simulink model "PID_Discrete"  (R2021b)
settings: Solver=VariableStepAuto  StartTime=0.0  StopTime=5  RelTol=1e-3  EnableMultiTasking=on
libraries: dspsrcs4 x3, simulink_extras x2, dspsigops x2, slpidlib x1, dsparch4 x1
settings Model: Creator=JelleKomen  LastModifiedBy=JelleKomen
settings DebuggingCC: SignalRangeChecking=warning

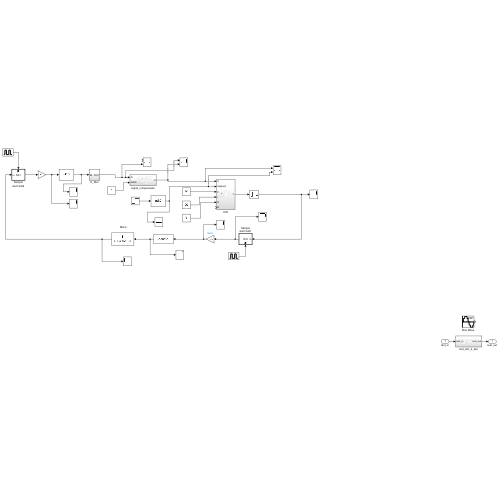
[thumbnail: Simulink's stored preview of the top-level diagram]
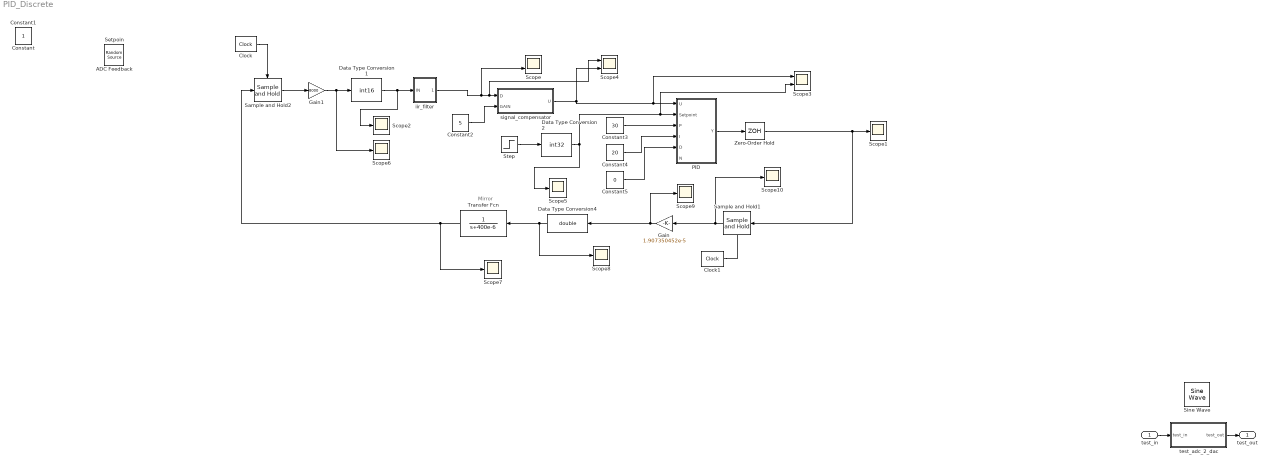
== system PID_Discrete ==
  note: Mirror
  test_in : Inport
  Clock : simulink_extras/Flip Flops/Clock  period=100e-9
  Clock1 : simulink_extras/Flip Flops/Clock  period=1e-6
  Constant2 : Constant  Value=5  OutDataTypeStr=uint8
  Constant3 : Constant  Value=30  OutDataTypeStr=int32
  Constant4 : Constant  Value=20  OutDataTypeStr=int32
  Constant5 : Constant  Value=0  OutDataTypeStr=int32
  Data Type Conversion1 : DataTypeConversion  OutDataTypeStr=int16
  Data Type Conversion2 : DataTypeConversion  OutDataTypeStr=int32
  Data Type Conversion4 : DataTypeConversion  OutDataTypeStr=double  SaturateOnIntegerOverflow=on
  Gain : Gain  Gain=1.907350452e-5
  Gain1 : Gain  Gain=8000
  PID : Subsystem
  Sample and Hold1 : dspsigops/Sample and Hold  trig=Rising edge  initCond=0  latchinput=off
  Sample and Hold2 : dspsigops/Sample and Hold  trig=Rising edge  initCond=0  latchinput=off
  Scope : Scope  NumInputPorts=2
  Scope{1..2,5..10} (8 alike) : Scope
  Scope3 : Scope  NumInputPorts=2
  Scope4 : Scope  NumInputPorts=2
  Sine Wave : dspsrcs4/Sine Wave  Amplitude=32767  Frequency=1e3  Phase=0  SampleMode=Discrete  OutComplex=Real  CompMethod=Table lookup  TableSize=Speed  SampleTime=1/10e6  SamplesPerFrame=1  ResetState=Restart at time zero  OutputFrames=off  dataType=Fixed-point  wordLen=16  udDataType=sfix(16)  fracBitsMode=User-defined  numFracBits=0  OutDataTypeStr=fixdt(1,16,0)  LastOutDataTypeStr=fixdt(1,16,0)
  Step : Step  Time=0.001  After=8000  SampleTime=0
  Transfer Fcn : TransferFcn  Denominator=[1 400e-6]
  Zero-Order Hold : ZeroOrderHold  SampleTime=-1
  iir_filter : Subsystem
  signal_compensator : Subsystem
  test_adc_2_dac : Subsystem
  test_out : Outport  VectorParamsAs1DForOutWhenUnconnected=off
  ADC Feedback : dspsrcs4/Random Source  IOType=siggen  SrcType=Uniform  NormMethod=Ziggurat  CltLength=12  MinVal=0  MaxVal=1  MeanVal=0  VarVal=1  RepMode=Not repeatable  rawSeed=1  IsInherit=off  SampMode=Discrete  SampTime=1  SampFrame=1  DataType=Double  OutComplex=Real  OutputFrames=on
  Constant : Constant  IOType=siggen
  Constant1 : Constant  IOType=siggen
  Setpoin : dspsrcs4/Random Source  IOType=siggen  SrcType=Uniform  NormMethod=Ziggurat  CltLength=12  MinVal=0  MaxVal=1  MeanVal=0  VarVal=1  RepMode=Not repeatable  rawSeed=1  IsInherit=off  SampMode=Discrete  SampTime=1  SampFrame=1  DataType=Double  OutComplex=Real  OutputFrames=on
  wires:
  test_in/1 -> test_adc_2_dac/1(test_in)
  test_adc_2_dac/1(test_out) -> test_out/1
  Constant2/1 -> signal_compensator/2(GAIN)
  signal_compensator/1(U) -> Scope4/2, PID/1(U), Scope3/1
  Zero-Order Hold/1 -> Sample and Hold1/1, Scope1/1
  Sample and Hold1/1 -> Gain/1, Scope10/1
  Clock1/1 -> Sample and Hold1/Trigger
  Data Type Conversion4/1 -> Transfer Fcn/1, Scope8/1
  PID/1(Y) -> Zero-Order Hold/1
  Step/1 -> Data Type Conversion2/1
  Data Type Conversion2/1 -> Scope5/1, PID/2(Setpoint), Scope3/2
  Constant3/1 -> PID/3(P)
  Gain/1 -> Scope9/1, Data Type Conversion4/1
  Constant4/1 -> PID/4(I)
  Transfer Fcn/1 -> Sample and Hold2/1, Scope7/1
  Constant5/1 -> PID/5(D)
  iir_filter/1(OUT) -> Scope/2, Scope4/1, signal_compensator/1(D)
  Gain1/1 -> Scope6/1, Data Type Conversion1/1
  Data Type Conversion1/1 -> Scope2/1, iir_filter/1(IN)
  Sample and Hold2/1 -> Gain1/1
  Clock/1 -> Sample and Hold2/Trigger

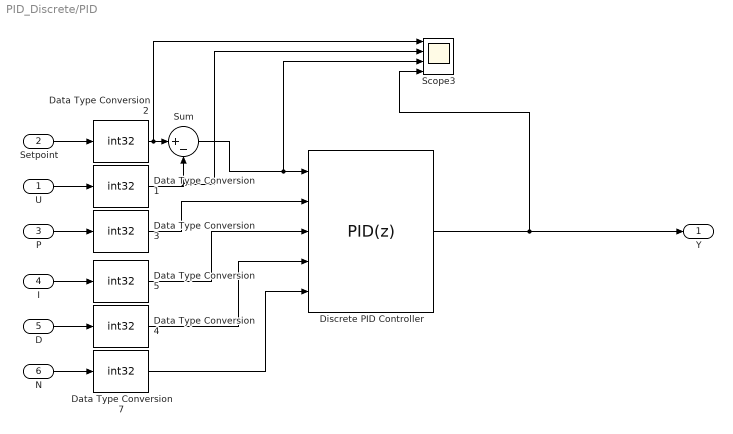
== system PID_Discrete/PID ==
  U : Inport  OutDataTypeStr=fixdt(1,20,0)
  Setpoint : Inport  Port=2  OutDataTypeStr=int32
  P : Inport  Port=3  OutDataTypeStr=int32
  I : Inport  Port=4  OutDataTypeStr=int32
  D : Inport  Port=5  OutDataTypeStr=int32
  N : Inport  Port=6  OutDataTypeStr=int32
  Data Type Conversion{1..5,7} (6 alike) : DataTypeConversion  OutDataTypeStr=int32  ConvertRealWorld=Stored Integer (SI)
  Discrete PID Controller : slpidlib/PID Controller  Controller=PID  Form=Parallel  TimeDomain=Discrete-time  UseExternalTs=off  SampleTime=-1  IntegratorMethod=Trapezoidal  FilterMethod=Forward Euler  ControllerParametersSource=external  P=1  I=1  D=0  UseFilter=on  N=100  TunerSelectOption=Transfer Function Based (PID Tuner App)  InitialConditionSource=internal  InitialConditionForIntegrator=0  InitialConditionForFilter=0  DifferentiatorICPrevScaledInput=0  ExternalReset=none  TrackingMode=off  Kt=1  LimitOutput=off  SatLimitsSource=internal  UpperSaturationLimit=inf  LowerSaturationLimit=-inf  LinearizeAsGain=off  AntiWindupMode=none  Kb=1  SaturateOnIntegerOverflow=on  PGainOutDataTypeStr=int32  PProdOutDataTypeStr=int32  POutMin=[]  POutMax=[]  IGainOutDataTypeStr=int32  IProdOutDataTypeStr=int32  IOutMin=[]  IOutMax=[]  DGainOutDataTypeStr=int32  DProdOutDataTypeStr=int32  DOutMin=[]  DOutMax=[]  NGainOutDataTypeStr=int32  NProdOutDataTypeStr=int32  NOutMin=[]  NOutMax=[]  SumOutDataTypeStr=int32  SumOutMin=[]  SumOutMax=[]  SaturationOutMin=[]  SaturationOutMax=[]  PParamMin=[]  PParamMax=[]  IParamMin=[]  IParamMax=[]  DParamMin=[]  DParamMax=[]  NParamMin=[]  NParamMax=[]  KbParamMin=[]  KbParamMax=[]  KtParamMin=[]  KtParamMax=[]  KbOutMin=[]  KbOutMax=[]  KtOutMin=[]  KtOutMax=[]  IntegratorOutDataTypeStr=int32  IntegratorOutMin=[]  IntegratorOutMax=[]  FilterOutDataTypeStr=int32  FilterOutMin=[]  FilterOutMax=[]  SumI1OutMin=[]  SumI1OutMax=[]  SumI2OutMin=[]  SumI2OutMax=[]  SumI3OutMin=[]  SumI3OutMax=[]  SumI4OutMin=[]  SumI4OutMax=[]  SumDOutDataTypeStr=int32  SumDOutMin=[]  SumDOutMax=[]  SumAccumDataTypeStr=int32  SumDAccumDataTypeStr=int32  DifferentiatorOutMin=[]  DifferentiatorOutMax=[]  FilterDiffOutCoefMin=[]  FilterDiffOutCoefMax=[]  ReciprocalOutMin=[]  ReciprocalOutMax=[]  SumDenOutMin=[]  SumDenOutMax=[]  SumNumOutMin=[]  SumNumOutMax=[]  DivideOutMin=[]  DivideOutMax=[]  UdiffTsProdOutMin=[]  UdiffTsProdOutMax=[]  NTsProdOutMin=[]  NTsProdOutMax=[]  UintegralTsProdOutMin=[]  UintegralTsProdOutMax=[]  UngainTsProdOutMin=[]  UngainTsProdOutMax=[]  IntegratorContinuousStateAttributes=''  IntegratorStateMustResolveToSignalObject=off  IntegratorRTWStateStorageClass=Auto  FilterContinuousStateAttributes=''  FilterStateMustResolveToSignalObject=off  FilterRTWStateStorageClass=Auto  ParallelPVariant=ExternalParameters  IdealPVariant=Disabled  IVariant=ExternalParameters  DVariant=ExternalParameters  IntegratorVariant=Discrete  SatVariant=Disabled  AWVariant=Passthrough  PCopyVariant=Disabled  TRVariant=Disabled  FdbkBlocksVariant=Forward  IdealPFdbkVariant=Disabled  SatFdbkVariant=Disabled  DerivativeFilterVariant=ForwardEulerFilter  NVariant=ExternalParameters  NCopyVariant=Disabled  FilterICVariant=InternalICsFilter  IntegratorICVariant=InternalICs  ExternalResetVariant=Disabled  TRSumVariant=Passthrough  SumFdbkVariant=Disabled  SumVariant=Sum_PID  TsampFilterVariant=InternalTs  TsampNgainVariant=Passthrough  TsampIntegralVariant=Passthrough  ExternalSaturationOutDataTypeStr=Inherit: Same as second input
      settings: LockScale=on
  Scope3 : Scope  NumInputPorts=4
  Sum : Sum  Inputs=|+-
  Y : Outport  OutDataTypeStr=fixdt(1,20,0)
  wires:
  U/1 -> Data Type Conversion1/1
  Data Type Conversion1/1 -> Scope3/2, Sum/2
  Data Type Conversion2/1 -> Scope3/1, Sum/1
  Setpoint/1 -> Data Type Conversion2/1
  P/1 -> Data Type Conversion3/1
  I/1 -> Data Type Conversion5/1
  D/1 -> Data Type Conversion4/1
  N/1 -> Data Type Conversion7/1
  Data Type Conversion3/1 -> Discrete PID Controller/2
  Data Type Conversion5/1 -> Discrete PID Controller/3
  Data Type Conversion4/1 -> Discrete PID Controller/4
  Data Type Conversion7/1 -> Discrete PID Controller/5
  Sum/1 -> Scope3/3, Discrete PID Controller/1
  Discrete PID Controller/1 -> Scope3/4, Y/1

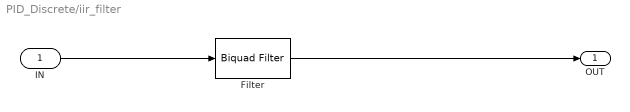
== system PID_Discrete/iir_filter ==
  IN : Inport  OutDataTypeStr=int16
  Filter : dsparch4/Biquad Filter  Tag=BlockMethodSubSystem  FilterSource=Dialog parameters  CoeffSource=Specify via dialog  FilterObject=BQF  IIRFiltStruct=Direct form II  BiQuadCoeffs=[1 2 1 1 -1.82450807943703452 0.904911483717982801;1 2 1 1 -1.67485327803320683 0.748661613958212513;1 2 1 1 -1.56987983878511672 0.639062148676173392;1 2 1 1 -1.50818165903315937 0.574645020323272693;1 1 0 1 -0.743936712675994705 0]  ScaleValues=[0.0201008510702371176;0.0184520839812514388;0.0172955774727642196;0.0166158403225283718;0.128031643662002703;1]  IC=0  ICnum=0  ICden=0  a0Flag=Warning  optimizeScaleValues=on  ScaleValueMode=Specify via input port (g)  InputProcessing=Columns as channels (frame based)  roundingMode=Floor  overflowMode=on  scaleValueFracLength=14  denProdOutputFracLength=30  denAccumFracLength=30  secondMemoryFracLength=15
  OUT : Outport  OutDataTypeStr=int16
  wires:
  IN/1 -> Filter/1
  Filter/1 -> OUT/1

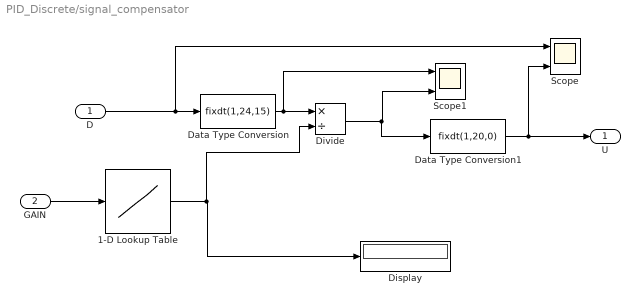
== system PID_Discrete/signal_compensator ==
  D : Inport  OutDataTypeStr=int16
  GAIN : Inport  Port=2  OutMin=0  OutMax=12  OutDataTypeStr=uint8
  1-D Lookup Table : Lookup_n-D  NumberOfTableDimensions=1  LookupTableObject=''  BreakpointsForDimension1=[1:12]  BreakpointsForDimension1FirstPoint=10  BreakpointsForDimension2FirstPoint=10  BreakpointsForDimension1Spacing=12  BreakpointsForDimension2Spacing=12  BreakpointsForDimension1DataTypeStr=uint8  IndexSearchMethod=Evenly spaced points  Table=[0.0625 0.125 0.25 0.5 1 2 4 8 16 32 64 128]  TableDataTypeStr=fixdt(1,24,15)  InterpMethod=Flat  DiagnosticForOutOfRangeInput=Error  OutDataTypeStr=fixdt(1,24,15)  RndMeth=Simplest  InputSameDT=on
  Data Type Conversion : DataTypeConversion  OutDataTypeStr=fixdt(1,24,15)  ConvertRealWorld=Stored Integer (SI)
  Data Type Conversion1 : DataTypeConversion  OutDataTypeStr=fixdt(1,20,0)  ConvertRealWorld=Stored Integer (SI)
  Display : Display
  Divide : Product  Inputs=*/  InputSameDT=on  OutDataTypeStr=fixdt(1,24,15)  RndMeth=Simplest  SaturateOnIntegerOverflow=on
  Scope : Scope  NumInputPorts=2
  Scope1 : Scope  NumInputPorts=2
  U : Outport
  wires:
  Divide/1 -> Data Type Conversion1/1, Scope1/2
  Data Type Conversion/1 -> Scope1/1, Divide/1
  1-D Lookup Table/1 -> Divide/2, Display/1
  Data Type Conversion1/1 -> U/1, Scope/2
  D/1 -> Scope/1, Data Type Conversion/1
  GAIN/1 -> 1-D Lookup Table/1

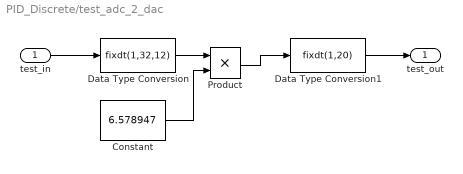
== system PID_Discrete/test_adc_2_dac ==
  test_in : Inport  OutMin=-32768  OutMax=32768  OutDataTypeStr=fixdt(1,16)
  Constant : Constant  Value=6.578947  OutDataTypeStr=fixdt(1,32,6)
  Data Type Conversion : DataTypeConversion  OutDataTypeStr=fixdt(1,32,12)
  Data Type Conversion1 : DataTypeConversion  OutMin=-524288  OutMax=524288  OutDataTypeStr=fixdt(1,20)
  Product : Product  OutDataTypeStr=fixdt(1,26,6)
  test_out : Outport
  wires:
  Data Type Conversion/1 -> Product/1
  Product/1 -> Data Type Conversion1/1
  Data Type Conversion1/1 -> test_out/1
  Constant/1 -> Product/2
  test_in/1 -> Data Type Conversion/1
